simulink model "UAV_Task3"  (R2024b)
settings: Solver=VariableStepAuto  StartTime=0  StopTime=200  RelTol=1e-5  AbsTol=1e-5
values from neighbouring files (symbols this model uses):
  adaptiveActivation = 1    [Simplified_UAV_Task3_main.m]    (also in newUAV_Task3_main.m)
  B_p = 1/UAV.m    [Simplified_UAV_Task3_main.m]    (also in newUAV_Task3_main.m)
  F2plus = F2'*pinv(F2*F2')    [Simplified_UAV_Task3_main.m]    (also in newUAV_Task3_main.m)
  Gamma_a = 1*[1 1 1 1]'    [Simplified_UAV_Task3_main.m]    (also in newUAV_Task3_main.m = 2*[1 1 1 1]')
  gravityInAdaptiveController = 1    [Simplified_UAV_Task3_main.m]    (also in newUAV_Task3_main.m)
  k_f = 0.3379e-6    (= 3.379e-07)    [Simplified_UAV_Task3_main.m]    (also in newUAV_Task3_main.m)
  L = 10    [Simplified_UAV_Task3_main.m]    (also in newUAV_Task3_main.m)
  lambda_0 = 1    [Simplified_UAV_Task3_main.m]    (also in newUAV_Task3_main.m)
  Omega_0 = [1500 1500 1500 1500]'    [Simplified_UAV_Task3_main.m]    (also in newUAV_Task3_main.m)
  omegab_0 = [0; 0; 0]    [Simplified_UAV_Task3_main.m]    (also in newUAV_Task3_main.m)
  p_0 = [0; 0; 0]    [Simplified_UAV_Task3_main.m]    (also in newUAV_Task3_main.m)
  PO = 1    [Simplified_UAV_Task3_main.m]    (also in newUAV_Task3_main.m)
  q_0 = eul2quat([0, 0, 0]*degToRad,'ZYX')'    [Simplified_UAV_Task3_main.m]    (also in newUAV_Task3_main.m)
  scenario = 2    [Simplified_UAV_Task3_main.m]    (also in newUAV_Task3_main.m)
  theta_0 = [0.07;0.07;0.1]    [Simplified_UAV_Task3_main.m]    (also in newUAV_Task3_main.m)
  vb_0 = [0; 0; 0]    [Simplified_UAV_Task3_main.m]    (also in newUAV_Task3_main.m)
undefined symbols (not defined in the file or in its folder): adaptive_controller, ctrl, D_fv_i, dyn, e_3, epsilon_PO, fw_params_fc, g, Gamma_a_scalar, lambda_i, par, pos, pos_pp, projection_operator, targetParams, theta_M, UAV, v_M, vel, vel_pp
libraries: slpidlib x22, matrix_library x6, aerolibutil x2, uavutilslib x1
(part 3 of 4)

== system UAV_Task3/Position Controller/Velocity controller (Dyn) ==
  e_v : Inport
  Demux : Demux  Outputs=3
  Mux : Mux  Inputs=3
  PID Controller vx : slpidlib/PID Controller  Controller=PI  Form=Parallel  TimeDomain=Continuous-time  UseExternalTs=off  SampleTime=-1  IntegratorMethod=Forward Euler  FilterMethod=Forward Euler  ControllerParametersSource=internal  P=ctrl.Kv(1,1)  I=ctrl.Kiv(1,1)  UseKiTs=off  D=0  UseExternalDerivativeSource=off  N=100  UseFilter=on  TunerSelectOption=Transfer Function Based (PID Tuner App)  InitialConditionSource=internal  InitialConditionForIntegrator=0  InitialConditionForFilter=0  DifferentiatorICPrevScaledInput=0  ExternalReset=none  TrackingMode=off  Kt=1  LimitOutput=off  SatLimitsSource=internal  UpperSaturationLimit=inf  LowerSaturationLimit=-inf  LinearizeAsGain=on  AntiWindupMode=none  Kb=1  LimitIntegrator=off  UpperIntegratorSaturationLimit=inf  LowerIntegratorSaturationLimit=-inf  POutMin=[]  POutMax=[]  IOutMin=[]  IOutMax=[]  DOutMin=[]  DOutMax=[]  NOutMin=[]  NOutMax=[]  SumOutMin=[]  SumOutMax=[]  SaturationOutMin=[]  SaturationOutMax=[]  PParamMin=[]  PParamMax=[]  IParamMin=[]  IParamMax=[]  DParamMin=[]  DParamMax=[]  NParamMin=[]  NParamMax=[]  KbParamMin=[]  KbParamMax=[]  KtParamMin=[]  KtParamMax=[]  KbOutMin=[]  KbOutMax=[]  KtOutMin=[]  KtOutMax=[]  IntegratorOutMin=[]  IntegratorOutMax=[]  FilterOutMin=[]  FilterOutMax=[]  SumI1OutMin=[]  SumI1OutMax=[]  SumI2OutMin=[]  SumI2OutMax=[]  SumI3OutMin=[]  SumI3OutMax=[]  SumI4OutMin=[]  SumI4OutMax=[]  SumDOutMin=[]  SumDOutMax=[]  DifferentiatorOutMin=[]  DifferentiatorOutMax=[]  FilterDiffOutCoefMin=[]  FilterDiffOutCoefMax=[]  ReciprocalOutMin=[]  ReciprocalOutMax=[]  SumDenOutMin=[]  SumDenOutMax=[]  SumNumOutMin=[]  SumNumOutMax=[]  DivideOutMin=[]  DivideOutMax=[]  UdiffTsProdOutMin=[]  UdiffTsProdOutMax=[]  NTsProdOutMin=[]  NTsProdOutMax=[]  UintegralTsProdOutMin=[]  UintegralTsProdOutMax=[]  UngainTsProdOutMin=[]  UngainTsProdOutMax=[]  ClampingZeroOutDataTypeStr=Inherit: Inherit via back propagation  ClampingZeroOutMin=[]  ClampingZeroOutMax=[]  FilterDenConstantOutDataTypeStr=Inherit: Inherit via back propagation  FilterDenConstantOutMin=[]  FilterDenConstantOutMax=[]  PCopyOutDataTypeStr=Inherit: Inherit via back propagation  PCopyOutMin=[]  PCopyOutMax=[]  NCopyOutDataTypeStr=Inherit: Inherit via back propagation  NCopyOutMin=[]  NCopyOutMax=[]  IntegratorContinuousStateAttributes=''  IntegratorStateMustResolveToSignalObject=off  IntegratorRTWStateStorageClass=Auto  FilterContinuousStateAttributes=''  FilterStateMustResolveToSignalObject=off  FilterRTWStateStorageClass=Auto  ParallelPVariant=InternalParameters  IdealPVariant=Disabled  IVariant=InternalParameters  DVariant=Disabled  IntegratorVariant=Continuous  SatVariant=Disabled  AWVariant=Passthrough  PCopyVariant=Disabled  TRVariant=Disabled  FdbkBlocksVariant=Forward  IdealPFdbkVariant=Disabled  SatFdbkVariant=Disabled  DerivativeFilterVariant=Disabled  NVariant=Disabled  NCopyVariant=Disabled_SignalSpec  FilterICVariant=Disabled  IntegratorICVariant=InternalICs  ExternalResetVariant=Disabled  TRSumVariant=Passthrough  SumFdbkVariant=Disabled  SumVariant=Sum_PI  TsampFilterVariant=InternalTs  TsampNgainVariant=Passthrough  TsampIntegralVariant=Disabled_SignalSpec  ExternalSaturationOutDataTypeStr=Inherit: Same as second input  DerivativeSourceVariant=Disabled  PreIntVariant=InternalPreInt
  PID Controller vy : slpidlib/PID Controller  Controller=PI  Form=Parallel  TimeDomain=Continuous-time  UseExternalTs=off  SampleTime=-1  IntegratorMethod=Forward Euler  FilterMethod=Forward Euler  ControllerParametersSource=internal  P=ctrl.Kv(2,2)  I=ctrl.Kiv(2,2)  UseKiTs=off  D=0  UseExternalDerivativeSource=off  N=100  UseFilter=on  TunerSelectOption=Transfer Function Based (PID Tuner App)  InitialConditionSource=internal  InitialConditionForIntegrator=0  InitialConditionForFilter=0  DifferentiatorICPrevScaledInput=0  ExternalReset=none  TrackingMode=off  Kt=1  LimitOutput=off  SatLimitsSource=internal  UpperSaturationLimit=inf  LowerSaturationLimit=-inf  LinearizeAsGain=on  AntiWindupMode=none  Kb=1  LimitIntegrator=off  UpperIntegratorSaturationLimit=inf  LowerIntegratorSaturationLimit=-inf  POutMin=[]  POutMax=[]  IOutMin=[]  IOutMax=[]  DOutMin=[]  DOutMax=[]  NOutMin=[]  NOutMax=[]  SumOutMin=[]  SumOutMax=[]  SaturationOutMin=[]  SaturationOutMax=[]  PParamMin=[]  PParamMax=[]  IParamMin=[]  IParamMax=[]  DParamMin=[]  DParamMax=[]  NParamMin=[]  NParamMax=[]  KbParamMin=[]  KbParamMax=[]  KtParamMin=[]  KtParamMax=[]  KbOutMin=[]  KbOutMax=[]  KtOutMin=[]  KtOutMax=[]  IntegratorOutMin=[]  IntegratorOutMax=[]  FilterOutMin=[]  FilterOutMax=[]  SumI1OutMin=[]  SumI1OutMax=[]  SumI2OutMin=[]  SumI2OutMax=[]  SumI3OutMin=[]  SumI3OutMax=[]  SumI4OutMin=[]  SumI4OutMax=[]  SumDOutMin=[]  SumDOutMax=[]  DifferentiatorOutMin=[]  DifferentiatorOutMax=[]  FilterDiffOutCoefMin=[]  FilterDiffOutCoefMax=[]  ReciprocalOutMin=[]  ReciprocalOutMax=[]  SumDenOutMin=[]  SumDenOutMax=[]  SumNumOutMin=[]  SumNumOutMax=[]  DivideOutMin=[]  DivideOutMax=[]  UdiffTsProdOutMin=[]  UdiffTsProdOutMax=[]  NTsProdOutMin=[]  NTsProdOutMax=[]  UintegralTsProdOutMin=[]  UintegralTsProdOutMax=[]  UngainTsProdOutMin=[]  UngainTsProdOutMax=[]  ClampingZeroOutDataTypeStr=Inherit: Inherit via back propagation  ClampingZeroOutMin=[]  ClampingZeroOutMax=[]  FilterDenConstantOutDataTypeStr=Inherit: Inherit via back propagation  FilterDenConstantOutMin=[]  FilterDenConstantOutMax=[]  PCopyOutDataTypeStr=Inherit: Inherit via back propagation  PCopyOutMin=[]  PCopyOutMax=[]  NCopyOutDataTypeStr=Inherit: Inherit via back propagation  NCopyOutMin=[]  NCopyOutMax=[]  IntegratorContinuousStateAttributes=''  IntegratorStateMustResolveToSignalObject=off  IntegratorRTWStateStorageClass=Auto  FilterContinuousStateAttributes=''  FilterStateMustResolveToSignalObject=off  FilterRTWStateStorageClass=Auto  ParallelPVariant=InternalParameters  IdealPVariant=Disabled  IVariant=InternalParameters  DVariant=Disabled  IntegratorVariant=Continuous  SatVariant=Disabled  AWVariant=Passthrough  PCopyVariant=Disabled  TRVariant=Disabled  FdbkBlocksVariant=Forward  IdealPFdbkVariant=Disabled  SatFdbkVariant=Disabled  DerivativeFilterVariant=Disabled  NVariant=Disabled  NCopyVariant=Disabled_SignalSpec  FilterICVariant=Disabled  IntegratorICVariant=InternalICs  ExternalResetVariant=Disabled  TRSumVariant=Passthrough  SumFdbkVariant=Disabled  SumVariant=Sum_PI  TsampFilterVariant=InternalTs  TsampNgainVariant=Passthrough  TsampIntegralVariant=Disabled_SignalSpec  ExternalSaturationOutDataTypeStr=Inherit: Same as second input  DerivativeSourceVariant=Disabled  PreIntVariant=InternalPreInt
  PID Controller vz : slpidlib/PID Controller  Controller=PI  Form=Parallel  TimeDomain=Continuous-time  UseExternalTs=off  SampleTime=-1  IntegratorMethod=Forward Euler  FilterMethod=Forward Euler  ControllerParametersSource=internal  P=ctrl.Kv(3,3)  I=ctrl.Kiv(3,3)  UseKiTs=off  D=0  UseExternalDerivativeSource=off  N=100  UseFilter=on  TunerSelectOption=Transfer Function Based (PID Tuner App)  InitialConditionSource=internal  InitialConditionForIntegrator=0  InitialConditionForFilter=0  DifferentiatorICPrevScaledInput=0  ExternalReset=none  TrackingMode=off  Kt=1  LimitOutput=off  SatLimitsSource=internal  UpperSaturationLimit=inf  LowerSaturationLimit=-inf  LinearizeAsGain=on  AntiWindupMode=none  Kb=1  LimitIntegrator=off  UpperIntegratorSaturationLimit=inf  LowerIntegratorSaturationLimit=-inf  POutMin=[]  POutMax=[]  IOutMin=[]  IOutMax=[]  DOutMin=[]  DOutMax=[]  NOutMin=[]  NOutMax=[]  SumOutMin=[]  SumOutMax=[]  SaturationOutMin=[]  SaturationOutMax=[]  PParamMin=[]  PParamMax=[]  IParamMin=[]  IParamMax=[]  DParamMin=[]  DParamMax=[]  NParamMin=[]  NParamMax=[]  KbParamMin=[]  KbParamMax=[]  KtParamMin=[]  KtParamMax=[]  KbOutMin=[]  KbOutMax=[]  KtOutMin=[]  KtOutMax=[]  IntegratorOutMin=[]  IntegratorOutMax=[]  FilterOutMin=[]  FilterOutMax=[]  SumI1OutMin=[]  SumI1OutMax=[]  SumI2OutMin=[]  SumI2OutMax=[]  SumI3OutMin=[]  SumI3OutMax=[]  SumI4OutMin=[]  SumI4OutMax=[]  SumDOutMin=[]  SumDOutMax=[]  DifferentiatorOutMin=[]  DifferentiatorOutMax=[]  FilterDiffOutCoefMin=[]  FilterDiffOutCoefMax=[]  ReciprocalOutMin=[]  ReciprocalOutMax=[]  SumDenOutMin=[]  SumDenOutMax=[]  SumNumOutMin=[]  SumNumOutMax=[]  DivideOutMin=[]  DivideOutMax=[]  UdiffTsProdOutMin=[]  UdiffTsProdOutMax=[]  NTsProdOutMin=[]  NTsProdOutMax=[]  UintegralTsProdOutMin=[]  UintegralTsProdOutMax=[]  UngainTsProdOutMin=[]  UngainTsProdOutMax=[]  ClampingZeroOutDataTypeStr=Inherit: Inherit via back propagation  ClampingZeroOutMin=[]  ClampingZeroOutMax=[]  FilterDenConstantOutDataTypeStr=Inherit: Inherit via back propagation  FilterDenConstantOutMin=[]  FilterDenConstantOutMax=[]  PCopyOutDataTypeStr=Inherit: Inherit via back propagation  PCopyOutMin=[]  PCopyOutMax=[]  NCopyOutDataTypeStr=Inherit: Inherit via back propagation  NCopyOutMin=[]  NCopyOutMax=[]  IntegratorContinuousStateAttributes=''  IntegratorStateMustResolveToSignalObject=off  IntegratorRTWStateStorageClass=Auto  FilterContinuousStateAttributes=''  FilterStateMustResolveToSignalObject=off  FilterRTWStateStorageClass=Auto  ParallelPVariant=InternalParameters  IdealPVariant=Disabled  IVariant=InternalParameters  DVariant=Disabled  IntegratorVariant=Continuous  SatVariant=Disabled  AWVariant=Passthrough  PCopyVariant=Disabled  TRVariant=Disabled  FdbkBlocksVariant=Forward  IdealPFdbkVariant=Disabled  SatFdbkVariant=Disabled  DerivativeFilterVariant=Disabled  NVariant=Disabled  NCopyVariant=Disabled_SignalSpec  FilterICVariant=Disabled  IntegratorICVariant=InternalICs  ExternalResetVariant=Disabled  TRSumVariant=Passthrough  SumFdbkVariant=Disabled  SumVariant=Sum_PI  TsampFilterVariant=InternalTs  TsampNgainVariant=Passthrough  TsampIntegralVariant=Disabled_SignalSpec  ExternalSaturationOutDataTypeStr=Inherit: Same as second input  DerivativeSourceVariant=Disabled  PreIntVariant=InternalPreInt
  2 : Outport
  wires:
  PID Controller vy/1 -> Mux/2
  Demux/2 -> PID Controller vy/1
  e_v/1 -> Demux/1
  Demux/3 -> PID Controller vz/1
  PID Controller vx/1 -> Mux/1
  PID Controller vz/1 -> Mux/3
  Demux/1 -> PID Controller vx/1
  Mux/1 -> 2/1

== system UAV_Task3/ATTITUDE CONTROLLER/Attitude dynamics FF/Feedback controller ==
  e_omega : Inport
  Demux : Demux  Outputs=3
  Mux : Mux  Inputs=3
  PID Controller p : slpidlib/PID Controller  Controller=PI  Form=Parallel  TimeDomain=Continuous-time  UseExternalTs=off  SampleTime=-1  IntegratorMethod=Forward Euler  FilterMethod=Forward Euler  ControllerParametersSource=internal  P=dyn.Kp(1,1)  I=dyn.Ki(1,1)  UseKiTs=off  D=0  UseExternalDerivativeSource=off  N=100  UseFilter=on  TunerSelectOption=Transfer Function Based (PID Tuner App)  InitialConditionSource=internal  InitialConditionForIntegrator=0  InitialConditionForFilter=0  DifferentiatorICPrevScaledInput=0  ExternalReset=none  TrackingMode=off  Kt=1  LimitOutput=off  SatLimitsSource=internal  UpperSaturationLimit=inf  LowerSaturationLimit=-inf  LinearizeAsGain=on  AntiWindupMode=none  Kb=1  LimitIntegrator=off  UpperIntegratorSaturationLimit=inf  LowerIntegratorSaturationLimit=-inf  POutMin=[]  POutMax=[]  IOutMin=[]  IOutMax=[]  DOutMin=[]  DOutMax=[]  NOutMin=[]  NOutMax=[]  SumOutMin=[]  SumOutMax=[]  SaturationOutMin=[]  SaturationOutMax=[]  PParamMin=[]  PParamMax=[]  IParamMin=[]  IParamMax=[]  DParamMin=[]  DParamMax=[]  NParamMin=[]  NParamMax=[]  KbParamMin=[]  KbParamMax=[]  KtParamMin=[]  KtParamMax=[]  KbOutMin=[]  KbOutMax=[]  KtOutMin=[]  KtOutMax=[]  IntegratorOutMin=[]  IntegratorOutMax=[]  FilterOutMin=[]  FilterOutMax=[]  SumI1OutMin=[]  SumI1OutMax=[]  SumI2OutMin=[]  SumI2OutMax=[]  SumI3OutMin=[]  SumI3OutMax=[]  SumI4OutMin=[]  SumI4OutMax=[]  SumDOutMin=[]  SumDOutMax=[]  DifferentiatorOutMin=[]  DifferentiatorOutMax=[]  FilterDiffOutCoefMin=[]  FilterDiffOutCoefMax=[]  ReciprocalOutMin=[]  ReciprocalOutMax=[]  SumDenOutMin=[]  SumDenOutMax=[]  SumNumOutMin=[]  SumNumOutMax=[]  DivideOutMin=[]  DivideOutMax=[]  UdiffTsProdOutMin=[]  UdiffTsProdOutMax=[]  NTsProdOutMin=[]  NTsProdOutMax=[]  UintegralTsProdOutMin=[]  UintegralTsProdOutMax=[]  UngainTsProdOutMin=[]  UngainTsProdOutMax=[]  ClampingZeroOutDataTypeStr=Inherit: Inherit via back propagation  ClampingZeroOutMin=[]  ClampingZeroOutMax=[]  FilterDenConstantOutDataTypeStr=Inherit: Inherit via back propagation  FilterDenConstantOutMin=[]  FilterDenConstantOutMax=[]  PCopyOutDataTypeStr=Inherit: Inherit via back propagation  PCopyOutMin=[]  PCopyOutMax=[]  NCopyOutDataTypeStr=Inherit: Inherit via back propagation  NCopyOutMin=[]  NCopyOutMax=[]  IntegratorContinuousStateAttributes=''  IntegratorStateMustResolveToSignalObject=off  IntegratorRTWStateStorageClass=Auto  FilterContinuousStateAttributes=''  FilterStateMustResolveToSignalObject=off  FilterRTWStateStorageClass=Auto  ParallelPVariant=InternalParameters  IdealPVariant=Disabled  IVariant=InternalParameters  DVariant=Disabled  IntegratorVariant=Continuous  SatVariant=Disabled  AWVariant=Passthrough  PCopyVariant=Disabled  TRVariant=Disabled  FdbkBlocksVariant=Forward  IdealPFdbkVariant=Disabled  SatFdbkVariant=Disabled  DerivativeFilterVariant=Disabled  NVariant=Disabled  NCopyVariant=Disabled_SignalSpec  FilterICVariant=Disabled  IntegratorICVariant=InternalICs  ExternalResetVariant=Disabled  TRSumVariant=Passthrough  SumFdbkVariant=Disabled  SumVariant=Sum_PI  TsampFilterVariant=InternalTs  TsampNgainVariant=Passthrough  TsampIntegralVariant=Disabled_SignalSpec  ExternalSaturationOutDataTypeStr=Inherit: Same as second input  DerivativeSourceVariant=Disabled  PreIntVariant=InternalPreInt
  PID Controller q : slpidlib/PID Controller  Controller=PI  Form=Parallel  TimeDomain=Continuous-time  UseExternalTs=off  SampleTime=-1  IntegratorMethod=Forward Euler  FilterMethod=Forward Euler  ControllerParametersSource=internal  P=dyn.Kp(2,2)  I=dyn.Ki(2,2)  UseKiTs=off  D=0  UseExternalDerivativeSource=off  N=100  UseFilter=on  TunerSelectOption=Transfer Function Based (PID Tuner App)  InitialConditionSource=internal  InitialConditionForIntegrator=0  InitialConditionForFilter=0  DifferentiatorICPrevScaledInput=0  ExternalReset=none  TrackingMode=off  Kt=1  LimitOutput=off  SatLimitsSource=internal  UpperSaturationLimit=inf  LowerSaturationLimit=-inf  LinearizeAsGain=on  AntiWindupMode=none  Kb=1  LimitIntegrator=off  UpperIntegratorSaturationLimit=inf  LowerIntegratorSaturationLimit=-inf  POutMin=[]  POutMax=[]  IOutMin=[]  IOutMax=[]  DOutMin=[]  DOutMax=[]  NOutMin=[]  NOutMax=[]  SumOutMin=[]  SumOutMax=[]  SaturationOutMin=[]  SaturationOutMax=[]  PParamMin=[]  PParamMax=[]  IParamMin=[]  IParamMax=[]  DParamMin=[]  DParamMax=[]  NParamMin=[]  NParamMax=[]  KbParamMin=[]  KbParamMax=[]  KtParamMin=[]  KtParamMax=[]  KbOutMin=[]  KbOutMax=[]  KtOutMin=[]  KtOutMax=[]  IntegratorOutMin=[]  IntegratorOutMax=[]  FilterOutMin=[]  FilterOutMax=[]  SumI1OutMin=[]  SumI1OutMax=[]  SumI2OutMin=[]  SumI2OutMax=[]  SumI3OutMin=[]  SumI3OutMax=[]  SumI4OutMin=[]  SumI4OutMax=[]  SumDOutMin=[]  SumDOutMax=[]  DifferentiatorOutMin=[]  DifferentiatorOutMax=[]  FilterDiffOutCoefMin=[]  FilterDiffOutCoefMax=[]  ReciprocalOutMin=[]  ReciprocalOutMax=[]  SumDenOutMin=[]  SumDenOutMax=[]  SumNumOutMin=[]  SumNumOutMax=[]  DivideOutMin=[]  DivideOutMax=[]  UdiffTsProdOutMin=[]  UdiffTsProdOutMax=[]  NTsProdOutMin=[]  NTsProdOutMax=[]  UintegralTsProdOutMin=[]  UintegralTsProdOutMax=[]  UngainTsProdOutMin=[]  UngainTsProdOutMax=[]  ClampingZeroOutDataTypeStr=Inherit: Inherit via back propagation  ClampingZeroOutMin=[]  ClampingZeroOutMax=[]  FilterDenConstantOutDataTypeStr=Inherit: Inherit via back propagation  FilterDenConstantOutMin=[]  FilterDenConstantOutMax=[]  PCopyOutDataTypeStr=Inherit: Inherit via back propagation  PCopyOutMin=[]  PCopyOutMax=[]  NCopyOutDataTypeStr=Inherit: Inherit via back propagation  NCopyOutMin=[]  NCopyOutMax=[]  IntegratorContinuousStateAttributes=''  IntegratorStateMustResolveToSignalObject=off  IntegratorRTWStateStorageClass=Auto  FilterContinuousStateAttributes=''  FilterStateMustResolveToSignalObject=off  FilterRTWStateStorageClass=Auto  ParallelPVariant=InternalParameters  IdealPVariant=Disabled  IVariant=InternalParameters  DVariant=Disabled  IntegratorVariant=Continuous  SatVariant=Disabled  AWVariant=Passthrough  PCopyVariant=Disabled  TRVariant=Disabled  FdbkBlocksVariant=Forward  IdealPFdbkVariant=Disabled  SatFdbkVariant=Disabled  DerivativeFilterVariant=Disabled  NVariant=Disabled  NCopyVariant=Disabled_SignalSpec  FilterICVariant=Disabled  IntegratorICVariant=InternalICs  ExternalResetVariant=Disabled  TRSumVariant=Passthrough  SumFdbkVariant=Disabled  SumVariant=Sum_PI  TsampFilterVariant=InternalTs  TsampNgainVariant=Passthrough  TsampIntegralVariant=Disabled_SignalSpec  ExternalSaturationOutDataTypeStr=Inherit: Same as second input  DerivativeSourceVariant=Disabled  PreIntVariant=InternalPreInt
  PID Controller r : slpidlib/PID Controller  Controller=PI  Form=Parallel  TimeDomain=Continuous-time  UseExternalTs=off  SampleTime=-1  IntegratorMethod=Forward Euler  FilterMethod=Forward Euler  ControllerParametersSource=internal  P=dyn.Kp(3,3)  I=dyn.Ki(3,3)  UseKiTs=off  D=0  UseExternalDerivativeSource=off  N=100  UseFilter=on  TunerSelectOption=Transfer Function Based (PID Tuner App)  InitialConditionSource=internal  InitialConditionForIntegrator=0  InitialConditionForFilter=0  DifferentiatorICPrevScaledInput=0  ExternalReset=none  TrackingMode=off  Kt=1  LimitOutput=off  SatLimitsSource=internal  UpperSaturationLimit=inf  LowerSaturationLimit=-inf  LinearizeAsGain=on  AntiWindupMode=none  Kb=1  LimitIntegrator=off  UpperIntegratorSaturationLimit=inf  LowerIntegratorSaturationLimit=-inf  POutMin=[]  POutMax=[]  IOutMin=[]  IOutMax=[]  DOutMin=[]  DOutMax=[]  NOutMin=[]  NOutMax=[]  SumOutMin=[]  SumOutMax=[]  SaturationOutMin=[]  SaturationOutMax=[]  PParamMin=[]  PParamMax=[]  IParamMin=[]  IParamMax=[]  DParamMin=[]  DParamMax=[]  NParamMin=[]  NParamMax=[]  KbParamMin=[]  KbParamMax=[]  KtParamMin=[]  KtParamMax=[]  KbOutMin=[]  KbOutMax=[]  KtOutMin=[]  KtOutMax=[]  IntegratorOutMin=[]  IntegratorOutMax=[]  FilterOutMin=[]  FilterOutMax=[]  SumI1OutMin=[]  SumI1OutMax=[]  SumI2OutMin=[]  SumI2OutMax=[]  SumI3OutMin=[]  SumI3OutMax=[]  SumI4OutMin=[]  SumI4OutMax=[]  SumDOutMin=[]  SumDOutMax=[]  DifferentiatorOutMin=[]  DifferentiatorOutMax=[]  FilterDiffOutCoefMin=[]  FilterDiffOutCoefMax=[]  ReciprocalOutMin=[]  ReciprocalOutMax=[]  SumDenOutMin=[]  SumDenOutMax=[]  SumNumOutMin=[]  SumNumOutMax=[]  DivideOutMin=[]  DivideOutMax=[]  UdiffTsProdOutMin=[]  UdiffTsProdOutMax=[]  NTsProdOutMin=[]  NTsProdOutMax=[]  UintegralTsProdOutMin=[]  UintegralTsProdOutMax=[]  UngainTsProdOutMin=[]  UngainTsProdOutMax=[]  ClampingZeroOutDataTypeStr=Inherit: Inherit via back propagation  ClampingZeroOutMin=[]  ClampingZeroOutMax=[]  FilterDenConstantOutDataTypeStr=Inherit: Inherit via back propagation  FilterDenConstantOutMin=[]  FilterDenConstantOutMax=[]  PCopyOutDataTypeStr=Inherit: Inherit via back propagation  PCopyOutMin=[]  PCopyOutMax=[]  NCopyOutDataTypeStr=Inherit: Inherit via back propagation  NCopyOutMin=[]  NCopyOutMax=[]  IntegratorContinuousStateAttributes=''  IntegratorStateMustResolveToSignalObject=off  IntegratorRTWStateStorageClass=Auto  FilterContinuousStateAttributes=''  FilterStateMustResolveToSignalObject=off  FilterRTWStateStorageClass=Auto  ParallelPVariant=InternalParameters  IdealPVariant=Disabled  IVariant=InternalParameters  DVariant=Disabled  IntegratorVariant=Continuous  SatVariant=Disabled  AWVariant=Passthrough  PCopyVariant=Disabled  TRVariant=Disabled  FdbkBlocksVariant=Forward  IdealPFdbkVariant=Disabled  SatFdbkVariant=Disabled  DerivativeFilterVariant=Disabled  NVariant=Disabled  NCopyVariant=Disabled_SignalSpec  FilterICVariant=Disabled  IntegratorICVariant=InternalICs  ExternalResetVariant=Disabled  TRSumVariant=Passthrough  SumFdbkVariant=Disabled  SumVariant=Sum_PI  TsampFilterVariant=InternalTs  TsampNgainVariant=Passthrough  TsampIntegralVariant=Disabled_SignalSpec  ExternalSaturationOutDataTypeStr=Inherit: Same as second input  DerivativeSourceVariant=Disabled  PreIntVariant=InternalPreInt
  tau_fbk : Outport
  wires:
  Mux/1 -> tau_fbk/1
  Demux/1 -> PID Controller p/1
  PID Controller r/1 -> Mux/3
  PID Controller p/1 -> Mux/1
  Demux/3 -> PID Controller r/1
  e_omega/1 -> Demux/1
  Demux/2 -> PID Controller q/1
  PID Controller q/1 -> Mux/2

== system UAV_Task3/POSITION + ADAPTIVE CONTROLLER/POSITION CONTROLLER/Position controller ==
  p : Inport
  p_d : Inport  Port=2
  v_d : Inport  Port=3
  a_d : Inport  Port=4
  v : Inport  Port=5
  MATLAB Function1 : MATLAB Function  TreatAsAtomicUnit=on
  " v_c" : Outport
  " a_c" : Outport  Port=2
  wires:
  MATLAB Function1/1(v_c) -> " v_c"/1
  a_d/1 -> MATLAB Function1/5(a_d)
  p/1 -> MATLAB Function1/1(p)
  p_d/1 -> MATLAB Function1/3(p_d)  "p_d"
  v_d/1 -> MATLAB Function1/4(v_d)
  v/1 -> MATLAB Function1/2(v)
  MATLAB Function1/2(a_c) -> " a_c"/1

== system UAV_Task3/POSITION + ADAPTIVE CONTROLLER/POSITION CONTROLLER/Velocity Controller ==
  v : Inport
  v_c : Inport  Port=2
  a_c : Inport  Port=3
  Demux : Demux  Outputs=3
  Gain : Gain  Gain=UAV.m
  Mux : Mux  Inputs=3
  PID Controller1 : slpidlib/PID Controller  Controller=PI  Form=Parallel  TimeDomain=Continuous-time  UseExternalTs=off  SampleTime=-1  IntegratorMethod=Forward Euler  FilterMethod=Forward Euler  ControllerParametersSource=internal  P=vel.Kp(2,2)  I=vel.Ki(2,2)  UseKiTs=off  D=0  UseExternalDerivativeSource=off  N=100  UseFilter=on  TunerSelectOption=Transfer Function Based (PID Tuner App)  InitialConditionSource=internal  InitialConditionForIntegrator=0  InitialConditionForFilter=0  DifferentiatorICPrevScaledInput=0  ExternalReset=none  TrackingMode=off  Kt=1  LimitOutput=off  SatLimitsSource=internal  UpperSaturationLimit=inf  LowerSaturationLimit=-inf  LinearizeAsGain=on  AntiWindupMode=none  Kb=1  LimitIntegrator=off  UpperIntegratorSaturationLimit=inf  LowerIntegratorSaturationLimit=-inf  POutMin=[]  POutMax=[]  IOutMin=[]  IOutMax=[]  DOutMin=[]  DOutMax=[]  NOutMin=[]  NOutMax=[]  SumOutMin=[]  SumOutMax=[]  SaturationOutMin=[]  SaturationOutMax=[]  PParamMin=[]  PParamMax=[]  IParamMin=[]  IParamMax=[]  DParamMin=[]  DParamMax=[]  NParamMin=[]  NParamMax=[]  KbParamMin=[]  KbParamMax=[]  KtParamMin=[]  KtParamMax=[]  KbOutMin=[]  KbOutMax=[]  KtOutMin=[]  KtOutMax=[]  IntegratorOutMin=[]  IntegratorOutMax=[]  FilterOutMin=[]  FilterOutMax=[]  SumI1OutMin=[]  SumI1OutMax=[]  SumI2OutMin=[]  SumI2OutMax=[]  SumI3OutMin=[]  SumI3OutMax=[]  SumI4OutMin=[]  SumI4OutMax=[]  SumDOutMin=[]  SumDOutMax=[]  DifferentiatorOutMin=[]  DifferentiatorOutMax=[]  FilterDiffOutCoefMin=[]  FilterDiffOutCoefMax=[]  ReciprocalOutMin=[]  ReciprocalOutMax=[]  SumDenOutMin=[]  SumDenOutMax=[]  SumNumOutMin=[]  SumNumOutMax=[]  DivideOutMin=[]  DivideOutMax=[]  UdiffTsProdOutMin=[]  UdiffTsProdOutMax=[]  NTsProdOutMin=[]  NTsProdOutMax=[]  UintegralTsProdOutMin=[]  UintegralTsProdOutMax=[]  UngainTsProdOutMin=[]  UngainTsProdOutMax=[]  ClampingZeroOutDataTypeStr=Inherit: Inherit via back propagation  ClampingZeroOutMin=[]  ClampingZeroOutMax=[]  FilterDenConstantOutDataTypeStr=Inherit: Inherit via back propagation  FilterDenConstantOutMin=[]  FilterDenConstantOutMax=[]  PCopyOutDataTypeStr=Inherit: Inherit via back propagation  PCopyOutMin=[]  PCopyOutMax=[]  NCopyOutDataTypeStr=Inherit: Inherit via back propagation  NCopyOutMin=[]  NCopyOutMax=[]  IntegratorContinuousStateAttributes=''  IntegratorStateMustResolveToSignalObject=off  IntegratorRTWStateStorageClass=Auto  FilterContinuousStateAttributes=''  FilterStateMustResolveToSignalObject=off  FilterRTWStateStorageClass=Auto  ParallelPVariant=InternalParameters  IdealPVariant=Disabled  IVariant=InternalParameters  DVariant=Disabled  IntegratorVariant=Continuous  SatVariant=Disabled  AWVariant=Passthrough  PCopyVariant=Disabled  TRVariant=Disabled  FdbkBlocksVariant=Forward  IdealPFdbkVariant=Disabled  SatFdbkVariant=Disabled  DerivativeFilterVariant=Disabled  NVariant=Disabled  NCopyVariant=Disabled_SignalSpec  FilterICVariant=Disabled  IntegratorICVariant=InternalICs  ExternalResetVariant=Disabled  TRSumVariant=Passthrough  SumFdbkVariant=Disabled  SumVariant=Sum_PI  TsampFilterVariant=InternalTs  TsampNgainVariant=Passthrough  TsampIntegralVariant=Disabled_SignalSpec  ExternalSaturationOutDataTypeStr=Inherit: Same as second input  DerivativeSourceVariant=Disabled  PreIntVariant=InternalPreInt
  PID Controller2 : slpidlib/PID Controller  Controller=PI  Form=Parallel  TimeDomain=Continuous-time  UseExternalTs=off  SampleTime=-1  IntegratorMethod=Forward Euler  FilterMethod=Forward Euler  ControllerParametersSource=internal  P=vel.Kp(3,3)  I=vel.Ki(3,3)  UseKiTs=off  D=0  UseExternalDerivativeSource=off  N=100  UseFilter=on  TunerSelectOption=Transfer Function Based (PID Tuner App)  InitialConditionSource=internal  InitialConditionForIntegrator=0  InitialConditionForFilter=0  DifferentiatorICPrevScaledInput=0  ExternalReset=none  TrackingMode=off  Kt=1  LimitOutput=off  SatLimitsSource=internal  UpperSaturationLimit=inf  LowerSaturationLimit=-inf  LinearizeAsGain=on  AntiWindupMode=none  Kb=1  LimitIntegrator=off  UpperIntegratorSaturationLimit=inf  LowerIntegratorSaturationLimit=-inf  POutMin=[]  POutMax=[]  IOutMin=[]  IOutMax=[]  DOutMin=[]  DOutMax=[]  NOutMin=[]  NOutMax=[]  SumOutMin=[]  SumOutMax=[]  SaturationOutMin=[]  SaturationOutMax=[]  PParamMin=[]  PParamMax=[]  IParamMin=[]  IParamMax=[]  DParamMin=[]  DParamMax=[]  NParamMin=[]  NParamMax=[]  KbParamMin=[]  KbParamMax=[]  KtParamMin=[]  KtParamMax=[]  KbOutMin=[]  KbOutMax=[]  KtOutMin=[]  KtOutMax=[]  IntegratorOutMin=[]  IntegratorOutMax=[]  FilterOutMin=[]  FilterOutMax=[]  SumI1OutMin=[]  SumI1OutMax=[]  SumI2OutMin=[]  SumI2OutMax=[]  SumI3OutMin=[]  SumI3OutMax=[]  SumI4OutMin=[]  SumI4OutMax=[]  SumDOutMin=[]  SumDOutMax=[]  DifferentiatorOutMin=[]  DifferentiatorOutMax=[]  FilterDiffOutCoefMin=[]  FilterDiffOutCoefMax=[]  ReciprocalOutMin=[]  ReciprocalOutMax=[]  SumDenOutMin=[]  SumDenOutMax=[]  SumNumOutMin=[]  SumNumOutMax=[]  DivideOutMin=[]  DivideOutMax=[]  UdiffTsProdOutMin=[]  UdiffTsProdOutMax=[]  NTsProdOutMin=[]  NTsProdOutMax=[]  UintegralTsProdOutMin=[]  UintegralTsProdOutMax=[]  UngainTsProdOutMin=[]  UngainTsProdOutMax=[]  ClampingZeroOutDataTypeStr=Inherit: Inherit via back propagation  ClampingZeroOutMin=[]  ClampingZeroOutMax=[]  FilterDenConstantOutDataTypeStr=Inherit: Inherit via back propagation  FilterDenConstantOutMin=[]  FilterDenConstantOutMax=[]  PCopyOutDataTypeStr=Inherit: Inherit via back propagation  PCopyOutMin=[]  PCopyOutMax=[]  NCopyOutDataTypeStr=Inherit: Inherit via back propagation  NCopyOutMin=[]  NCopyOutMax=[]  IntegratorContinuousStateAttributes=''  IntegratorStateMustResolveToSignalObject=off  IntegratorRTWStateStorageClass=Auto  FilterContinuousStateAttributes=''  FilterStateMustResolveToSignalObject=off  FilterRTWStateStorageClass=Auto  ParallelPVariant=InternalParameters  IdealPVariant=Disabled  IVariant=InternalParameters  DVariant=Disabled  IntegratorVariant=Continuous  SatVariant=Disabled  AWVariant=Passthrough  PCopyVariant=Disabled  TRVariant=Disabled  FdbkBlocksVariant=Forward  IdealPFdbkVariant=Disabled  SatFdbkVariant=Disabled  DerivativeFilterVariant=Disabled  NVariant=Disabled  NCopyVariant=Disabled_SignalSpec  FilterICVariant=Disabled  IntegratorICVariant=InternalICs  ExternalResetVariant=Disabled  TRSumVariant=Passthrough  SumFdbkVariant=Disabled  SumVariant=Sum_PI  TsampFilterVariant=InternalTs  TsampNgainVariant=Passthrough  TsampIntegralVariant=Disabled_SignalSpec  ExternalSaturationOutDataTypeStr=Inherit: Same as second input  DerivativeSourceVariant=Disabled  PreIntVariant=InternalPreInt
  PID Controller3 : slpidlib/PID Controller  Controller=PI  Form=Parallel  TimeDomain=Continuous-time  UseExternalTs=off  SampleTime=-1  IntegratorMethod=Forward Euler  FilterMethod=Forward Euler  ControllerParametersSource=internal  P=vel.Kp(1,1)  I=vel.Ki(1,1)  UseKiTs=off  D=0  UseExternalDerivativeSource=off  N=100  UseFilter=on  TunerSelectOption=Transfer Function Based (PID Tuner App)  InitialConditionSource=internal  InitialConditionForIntegrator=0  InitialConditionForFilter=0  DifferentiatorICPrevScaledInput=0  ExternalReset=none  TrackingMode=off  Kt=1  LimitOutput=off  SatLimitsSource=internal  UpperSaturationLimit=inf  LowerSaturationLimit=-inf  LinearizeAsGain=on  AntiWindupMode=none  Kb=1  LimitIntegrator=off  UpperIntegratorSaturationLimit=inf  LowerIntegratorSaturationLimit=-inf  POutMin=[]  POutMax=[]  IOutMin=[]  IOutMax=[]  DOutMin=[]  DOutMax=[]  NOutMin=[]  NOutMax=[]  SumOutMin=[]  SumOutMax=[]  SaturationOutMin=[]  SaturationOutMax=[]  PParamMin=[]  PParamMax=[]  IParamMin=[]  IParamMax=[]  DParamMin=[]  DParamMax=[]  NParamMin=[]  NParamMax=[]  KbParamMin=[]  KbParamMax=[]  KtParamMin=[]  KtParamMax=[]  KbOutMin=[]  KbOutMax=[]  KtOutMin=[]  KtOutMax=[]  IntegratorOutMin=[]  IntegratorOutMax=[]  FilterOutMin=[]  FilterOutMax=[]  SumI1OutMin=[]  SumI1OutMax=[]  SumI2OutMin=[]  SumI2OutMax=[]  SumI3OutMin=[]  SumI3OutMax=[]  SumI4OutMin=[]  SumI4OutMax=[]  SumDOutMin=[]  SumDOutMax=[]  DifferentiatorOutMin=[]  DifferentiatorOutMax=[]  FilterDiffOutCoefMin=[]  FilterDiffOutCoefMax=[]  ReciprocalOutMin=[]  ReciprocalOutMax=[]  SumDenOutMin=[]  SumDenOutMax=[]  SumNumOutMin=[]  SumNumOutMax=[]  DivideOutMin=[]  DivideOutMax=[]  UdiffTsProdOutMin=[]  UdiffTsProdOutMax=[]  NTsProdOutMin=[]  NTsProdOutMax=[]  UintegralTsProdOutMin=[]  UintegralTsProdOutMax=[]  UngainTsProdOutMin=[]  UngainTsProdOutMax=[]  ClampingZeroOutDataTypeStr=Inherit: Inherit via back propagation  ClampingZeroOutMin=[]  ClampingZeroOutMax=[]  FilterDenConstantOutDataTypeStr=Inherit: Inherit via back propagation  FilterDenConstantOutMin=[]  FilterDenConstantOutMax=[]  PCopyOutDataTypeStr=Inherit: Inherit via back propagation  PCopyOutMin=[]  PCopyOutMax=[]  NCopyOutDataTypeStr=Inherit: Inherit via back propagation  NCopyOutMin=[]  NCopyOutMax=[]  IntegratorContinuousStateAttributes=''  IntegratorStateMustResolveToSignalObject=off  IntegratorRTWStateStorageClass=Auto  FilterContinuousStateAttributes=''  FilterStateMustResolveToSignalObject=off  FilterRTWStateStorageClass=Auto  ParallelPVariant=InternalParameters  IdealPVariant=Disabled  IVariant=InternalParameters  DVariant=Disabled  IntegratorVariant=Continuous  SatVariant=Disabled  AWVariant=Passthrough  PCopyVariant=Disabled  TRVariant=Disabled  FdbkBlocksVariant=Forward  IdealPFdbkVariant=Disabled  SatFdbkVariant=Disabled  DerivativeFilterVariant=Disabled  NVariant=Disabled  NCopyVariant=Disabled_SignalSpec  FilterICVariant=Disabled  IntegratorICVariant=InternalICs  ExternalResetVariant=Disabled  TRSumVariant=Passthrough  SumFdbkVariant=Disabled  SumVariant=Sum_PI  TsampFilterVariant=InternalTs  TsampNgainVariant=Passthrough  TsampIntegralVariant=Disabled_SignalSpec  ExternalSaturationOutDataTypeStr=Inherit: Same as second input  DerivativeSourceVariant=Disabled  PreIntVariant=InternalPreInt
  Sum : Sum  Inputs=+-
  Sum1 : Sum  Inputs=--+
  "gravity compensation " : Constant  Value=UAV.m*g*e_3
  f_c : Outport
  wires:
  Demux/1 -> PID Controller3/1
  PID Controller1/1 -> Mux/2
  Demux/2 -> PID Controller1/1
  PID Controller2/1 -> Mux/3
  PID Controller3/1 -> Mux/1
  Sum/1 -> Demux/1  "e_v"
  Demux/3 -> PID Controller2/1
  v/1 -> Sum/1
  v_c/1 -> Sum/2
  a_c/1 -> Gain/1
  Sum1/1 -> f_c/1
  Mux/1 -> Sum1/2
  Gain/1 -> Sum1/3
  "gravity compensation "/1 -> Sum1/1

== system UAV_Task3/POSITION + ADAPTIVE CONTROLLER/Subsystem1/Subsystem ==
  v : Inport
  phipT : Inport  Port=2
  lambda_hat : Inport  Port=3
  u : Inport  Port=4
  thetap_hat : Inport  Port=5
  Constant : Constant  Value=[0 0 g]
  Gain : Gain  Gain=1/UAV.m
  Gain1 : Gain  Gain=L
  Integrator : Integrator  InitialCondition=vb_0
  Matrix Multiply : Product  Multiplication=Matrix(*)
  Matrix Multiply1 : Product  Multiplication=Matrix(*)
  Scope : Scope
  Sum : Sum  Inputs=+++
  Sum1 : Sum
  Sum2 : Sum  Inputs=|+-
  v_hat : Outport
  ev : Outport  Port=2
  wires:
  lambda_hat/1 -> Matrix Multiply/1
  u/1 -> Matrix Multiply/2
  phipT/1 -> Matrix Multiply1/1
  thetap_hat/1 -> Matrix Multiply1/2
  Matrix Multiply1/1 -> Sum1/1
  Matrix Multiply/1 -> Sum1/2
  Sum1/1 -> Gain/1
  Constant/1 -> Sum/1
  Gain/1 -> Sum/2
  Sum/1 -> Integrator/1
  Integrator/1 -> Sum2/2, v_hat/1
  v/1 -> Sum2/1
  Sum2/1 -> Scope/1, ev/1, Gain1/1
  Gain1/1 -> Sum/3

== system UAV_Task3/POSITION + ADAPTIVE CONTROLLER/Subsystem1/Subsystem1 ==
  phia : Inport
  ev : Inport  Port=2
  Adaptive Augmentation : Subsystem  Commented=on
  Constant : Constant  Value=Gamma_a_scalar
  Constant1 : Constant  Value=projection_operator
  Gain : Gain  Gain=1/UAV.m
  Integrator : Integrator  InitialCondition=[lambda_i; D_fv_i']
  Integrator1 : Integrator  InitialCondition=[lambda_i; D_fv_i']
  Matrix Multiply : Product
  Matrix Multiply1 : Product  Multiplication=Matrix(*)
  Projection operator : MATLAB Function  Commented=on  TreatAsAtomicUnit=on
  Scope : Scope
  Scope1 : Scope
  Switch : Switch  Criteria=u2 > Threshold  Threshold=0.5  SaturateOnIntegerOverflow=off  InputSameDT=off
  theta_a : Outport
  wires:
  Constant/1 -> Gain/1
  Gain/1 -> Matrix Multiply/1
  phia/1 -> Matrix Multiply/2
  Matrix Multiply/1 -> Matrix Multiply1/1
  ev/1 -> Matrix Multiply1/2
  Matrix Multiply1/1 -> Integrator/1, Projection operator/2(y)
  Integrator/1 -> Switch/3
  Projection operator/2(y_proj) -> Integrator1/1
  Integrator1/1 -> Projection operator/1(theta_a_hat), Switch/1
  Constant1/1 -> Switch/2
  Switch/1 -> theta_a/1
  Projection operator/1(f) -> Scope/1
  Projection operator/3(ygrad) -> Scope1/1

== system UAV_Task3/POSITION + ADAPTIVE CONTROLLER/Subsystem1/Subsystem2 ==
  lambda_mx : Inport
  ub : Inport  Port=2
  phipT : Inport  Port=3
  thetap_hat : Inport  Port=4
  Constant : Constant  Value=eye(3)
  Invert 3x3 Matrix : aerolibutil/Invert  3x3 Matrix
  Matrix Multiply : Product  Multiplication=Matrix(*)
  Matrix Multiply1 : Product  Multiplication=Matrix(*)
  Matrix Multiply2 : Product  Multiplication=Matrix(*)
  Sum : Sum  Inputs=|+-
  Sum1 : Sum  Inputs=+-
  ua : Outport
  wires:
  lambda_mx/1 -> Invert 3x3 Matrix/1
  Invert 3x3 Matrix/1 -> Matrix Multiply1/1, Sum/1
  Constant/1 -> Sum/2
  Sum/1 -> Matrix Multiply/1
  ub/1 -> Matrix Multiply/2
  Matrix Multiply/1 -> Sum1/1
  phipT/1 -> Matrix Multiply1/2
  Matrix Multiply1/1 -> Matrix Multiply2/1
  thetap_hat/1 -> Matrix Multiply2/2
  Matrix Multiply2/1 -> Sum1/2
  Sum1/1 -> ua/1

== system UAV_Task3/Position Controller/Adaptive Augmentation/Predictor (x_p_hat) dynamics ==
  Lambda_hat : Inport
  u : Inport  Port=2
  phi_p : Inport  Port=3
  theta_p_hat : Inport  Port=4
  x_p : Inport  Port=5
  Add : Sum
  Constant : Constant  Value=par.g*par.e_3
  Gain : Gain  Gain=B_p  Multiplication=Matrix(K*u)
  Gain1 : Gain  Gain=L
  Gain2 : Gain  Gain=gravityInAdaptiveController
  Gain3 : Gain
  Integrator : Integrator  InitialCondition=vb_0
  Matrix Multiply : Product
  Matrix Multiply1 : Product  Multiplication=Matrix(*)
  Reshape : Reshape  OutputDimensionality=Column vector (2-D)
  Reshape1 : Reshape  OutputDimensionality=Column vector (2-D)
  Reshape2 : Reshape  OutputDimensionality=Column vector (2-D)
  Scope : Scope
  Scope1 : Scope
  Sum : Sum  Inputs=+++
  Sum1 : Sum  Inputs=-+|
  Transpose : Math  Operator=transpose
  x_p_hat : Outport
  wires:
  Lambda_hat/1 -> Matrix Multiply/1
  phi_p/1 -> Transpose/1
  theta_p_hat/1 -> Matrix Multiply1/2
  Gain/1 -> Reshape1/1
  Gain1/1 -> Reshape/1
  x_p/1 -> Scope1/1, Sum1/2
  Sum1/1 -> Gain1/1
  Integrator/1 -> Scope/1, Sum1/1, x_p_hat/1
  Reshape/1 -> Sum/1  "prediction_error"
  Reshape1/1 -> Sum/2  "dynamics"
  Reshape2/1 -> Sum/3  "gravity"
  Constant/1 -> Gain2/1
  Transpose/1 -> Matrix Multiply1/1
  u/1 -> Matrix Multiply/2
  Gain2/1 -> Gain3/1
  Gain3/1 -> Reshape2/1
  Matrix Multiply1/1 -> Add/2
  Add/1 -> Gain/1
  Matrix Multiply/1 -> Add/1
  Sum/1 -> Integrator/1

== system UAV_Task3/Position Controller/Adaptive Augmentation/Subsystem ==
  Lambda_hat : Inport
  u_b : Inport  Port=2
  phi_p : Inport  Port=3
  theta_p_hat : Inport  Port=4
  Constant : Constant  Value=eye(3,3)
  Gain : Gain  Commented=through  Gain=-1
  Gain1 : Gain
  Inverse : MATLAB Function  TreatAsAtomicUnit=on
  Product : Product  Multiplication=Matrix(*)
  Product1 : Product  Inputs=3  Multiplication=Matrix(*)
  Subtract : Sum  Inputs=-+
  Subtract1 : Sum  Inputs=+-
  Transpose : Math  Operator=transpose
  u_a : Outport
  wires:
  Lambda_hat/1 -> Inverse/1(u)
  Inverse/1(y) -> Product1/1, Subtract/2
  Constant/1 -> Subtract/1
  Subtract/1 -> Product/1
  u_b/1 -> Product/2
  Product/1 -> Gain1/1
  Subtract1/1 -> u_a/1
  phi_p/1 -> Transpose/1
  Transpose/1 -> Gain/1
  theta_p_hat/1 -> Product1/3
  Product1/1 -> Subtract1/2
  Gain/1 -> Product1/2
  Gain1/1 -> Subtract1/1

== system UAV_Task3/Position Controller/Adaptive Augmentation/phi_a ==
  u : Inport
  phi_p : Inport  Port=2
  Matrix Concatenate : Concatenate  Mode=Multidimensional array
  Scope : Scope
  Transpose : Math  Operator=transpose
  phi_a : Outport
  wires:
  Matrix Concatenate/1 -> Scope/1, phi_a/1
  u/1 -> Transpose/1
  phi_p/1 -> Matrix Concatenate/2
  Transpose/1 -> Matrix Concatenate/1

== system UAV_Task3/Position Controller/Adaptive Augmentation/phi_p ==
  x_p : Inport
  Create Diagonal Matrix : matrix_library/Create Diagonal Matrix
  Gain : Gain  Gain=-1
  phi_p : Outport
  wires:
  x_p/1 -> Gain/1
  Gain/1 -> Create Diagonal Matrix/1
  Create Diagonal Matrix/1 -> phi_p/1

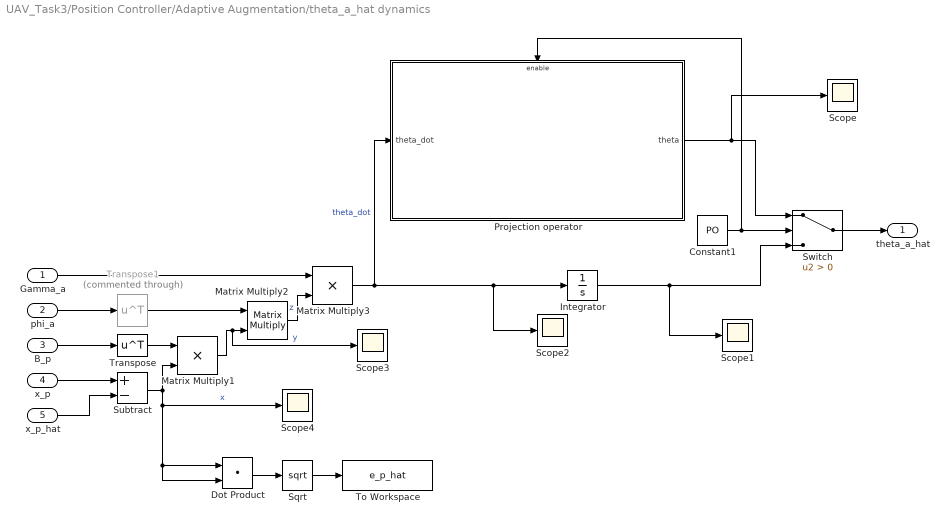
== system UAV_Task3/Position Controller/Adaptive Augmentation/theta_a_hat dynamics ==
  Gamma_a : Inport
  phi_a : Inport  Port=2
  B_p : Inport  Port=3
  x_p : Inport  Port=4
  x_p_hat : Inport  Port=5
  Constant1 : Constant  Value=PO
  Dot Product : DotProduct  OutDataTypeStr=Inherit: Inherit via internal rule
  Integrator : Integrator  InitialCondition=[lambda_0; theta_0]
  Matrix Multiply1 : Product
  Matrix Multiply2 : Product  Multiplication=Matrix(*)
  Matrix Multiply3 : Product
  Projection operator : Subsystem
  Scope{,1..4} (5 alike) : Scope
  Sqrt : Sqrt
  Subtract : Sum  Inputs=+-
  Switch : Switch  Criteria=u2 > Threshold  SaturateOnIntegerOverflow=off  InputSameDT=off
  To Workspace : ToWorkspace  VariableName=e_p_hat  SaveFormat=Timeseries  SampleTime=-1
  Transpose : Math  Operator=transpose
  Transpose1 : Math  Commented=through  Operator=transpose
  theta_a_hat : Outport
  wires:
  x_p_hat/1 -> Subtract/2
  B_p/1 -> Transpose/1
  Subtract/1 -> Scope4/1, Dot Product/2, Dot Product/1, Matrix Multiply1/2  "x"
  Transpose/1 -> Matrix Multiply1/1
  phi_a/1 -> Transpose1/1
  Matrix Multiply1/1 -> Scope3/1, Matrix Multiply2/2  "y"
  Gamma_a/1 -> Matrix Multiply3/1
  Matrix Multiply2/1 -> Matrix Multiply3/2  "z"
  Matrix Multiply3/1 -> Projection operator/1(theta_dot), Scope2/1, Integrator/1  "theta_dot"
  x_p/1 -> Subtract/1
  Constant1/1 -> Switch/2, Projection operator/Enable
  Integrator/1 -> Scope1/1, Switch/3
  Switch/1 -> theta_a_hat/1
  Projection operator/1(theta) -> Scope/1, Switch/1
  Dot Product/1 -> Sqrt/1
  Sqrt/1 -> To Workspace/1
  Transpose1/1 -> Matrix Multiply2/1

== system UAV_Task3/Position Controller/Position controller (Kin)/Subsystem ==
  e_p : Inport
  Action Port : ActionPort  ActionPortLabel=if(u1 == 2)
  Dot Product : DotProduct  OutDataTypeStr=Inherit: Inherit via internal rule
  Sqrt : Sqrt
  Sum of Elements : Sum  Inputs=+
  To Workspace : ToWorkspace  VariableName=posRMS  SaveFormat=Timeseries  SampleTime=-1
  wires:
  e_p/1 -> Dot Product/2, Dot Product/1
  Dot Product/1 -> Sum of Elements/1
  Sum of Elements/1 -> Sqrt/1
  Sqrt/1 -> To Workspace/1

== system UAV_Task3/Position Controller/Subsystem1/Subsystem ==
  v : Inport
  phipT : Inport  Port=2
  lambda_hat : Inport  Port=3
  u : Inport  Port=4
  thetap_hat : Inport  Port=5
  Constant : Constant  Value=[0 0 g]
  Gain : Gain  Gain=1/UAV.m
  Gain1 : Gain  Gain=L
  Integrator : Integrator  InitialCondition=vb_0
  Matrix Multiply : Product  Multiplication=Matrix(*)
  Matrix Multiply1 : Product  Multiplication=Matrix(*)
  Sum : Sum  Inputs=+++
  Sum1 : Sum
  Sum2 : Sum  Inputs=|+-
  v_hat : Outport
  ev : Outport  Port=2
  wires:
  lambda_hat/1 -> Matrix Multiply/1
  u/1 -> Matrix Multiply/2
  phipT/1 -> Matrix Multiply1/1
  thetap_hat/1 -> Matrix Multiply1/2
  Matrix Multiply1/1 -> Sum1/1
  Matrix Multiply/1 -> Sum1/2
  Sum1/1 -> Gain/1
  Constant/1 -> Sum/1
  Gain/1 -> Sum/2
  Sum/1 -> Integrator/1
  Integrator/1 -> Sum2/2, v_hat/1
  v/1 -> Sum2/1
  Sum2/1 -> ev/1, Gain1/1
  Gain1/1 -> Sum/3

== system UAV_Task3/Position Controller/Subsystem1/Subsystem1 ==
  phia : Inport
  ev : Inport  Port=2
  Constant : Constant  Value=Gamma_a_scalar
  Constant1 : Constant  Value=projection_operator
  Gain : Gain  Gain=1/UAV.m
  Integrator : Integrator  InitialCondition=[lambda_i; D_fv_i']
  Integrator1 : Integrator  InitialCondition=[lambda_i; D_fv_i']
  Matrix Multiply : Product
  Matrix Multiply1 : Product  Multiplication=Matrix(*)
  Projection operator : MATLAB Function  Commented=on  TreatAsAtomicUnit=on
  Reshape : Reshape  OutputDimensionality=Column vector (2-D)
  Scope : Scope
  Scope1 : Scope
  Switch : Switch  Criteria=u2 > Threshold  Threshold=0.5  SaturateOnIntegerOverflow=off  InputSameDT=off
  theta_a : Outport
  wires:
  Constant/1 -> Reshape/1
  Gain/1 -> Matrix Multiply/1
  phia/1 -> Matrix Multiply/2
  Matrix Multiply/1 -> Matrix Multiply1/1
  ev/1 -> Matrix Multiply1/2
  Matrix Multiply1/1 -> Integrator/1, Projection operator/2(y)
  Integrator/1 -> Switch/3
  Projection operator/2(y_proj) -> Integrator1/1
  Integrator1/1 -> Projection operator/1(theta_a_hat), Switch/1
  Constant1/1 -> Switch/2
  Switch/1 -> theta_a/1
  Projection operator/1(f) -> Scope/1
  Projection operator/3(ygrad) -> Scope1/1
  Reshape/1 -> Gain/1

== system UAV_Task3/Position Controller/Subsystem1/Subsystem2 ==
  lambda_mx : Inport
  ub : Inport  Port=2
  phipT : Inport  Port=3
  thetap_hat : Inport  Port=4
  Constant : Constant  Value=eye(3)
  Invert 3x3 Matrix : aerolibutil/Invert  3x3 Matrix
  Matrix Multiply : Product  Multiplication=Matrix(*)
  Matrix Multiply1 : Product  Multiplication=Matrix(*)
  Matrix Multiply2 : Product  Multiplication=Matrix(*)
  Sum : Sum  Inputs=|+-
  Sum1 : Sum  Inputs=+-
  ua : Outport
  wires:
  lambda_mx/1 -> Invert 3x3 Matrix/1
  Invert 3x3 Matrix/1 -> Matrix Multiply1/1, Sum/1
  Constant/1 -> Sum/2
  Sum/1 -> Matrix Multiply/1
  ub/1 -> Matrix Multiply/2
  Matrix Multiply/1 -> Sum1/1
  phipT/1 -> Matrix Multiply1/2
  Matrix Multiply1/1 -> Matrix Multiply2/1
  thetap_hat/1 -> Matrix Multiply2/2
  Matrix Multiply2/1 -> Sum1/2
  Sum1/1 -> ua/1

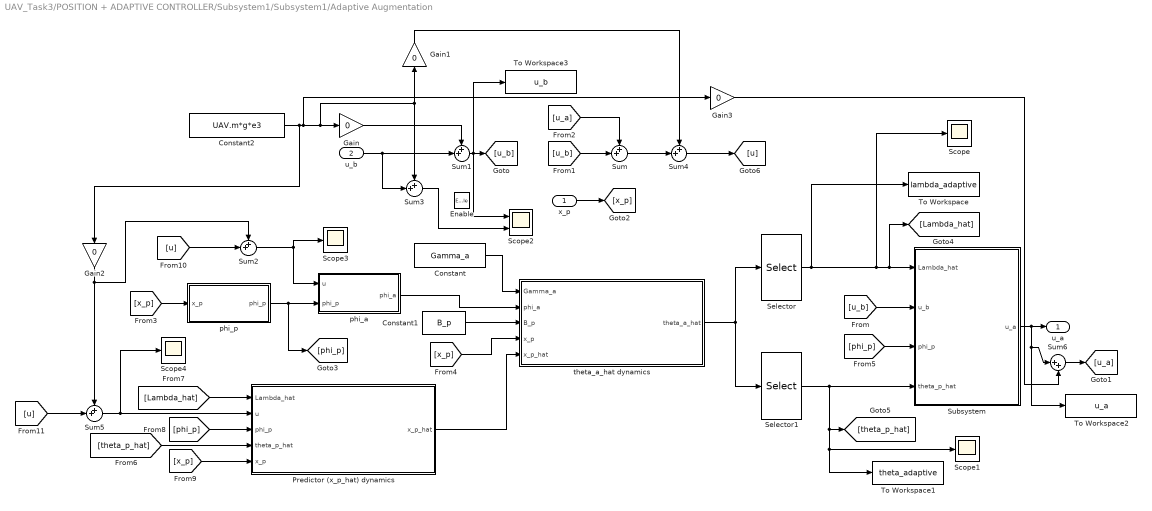
== system UAV_Task3/POSITION + ADAPTIVE CONTROLLER/Subsystem1/Subsystem1/Adaptive Augmentation ==
  x_p : Inport
  u_b : Inport  Port=2
  Enable : EnablePort
  Constant : Constant  Value=Gamma_a
  Constant1 : Constant  Value=B_p
  Constant2 : Constant  Value=UAV.m*g*e3
  Gain{,1..3} (4 alike) : Gain  Gain=0
  Predictor (x_p_hat) dynamics : Subsystem
  Scope{,1,3..4} (4 alike) : Scope
  Scope2 : Scope  NumInputPorts=2
  Selector : Selector  InputPortWidth=4  IndexOptions=Index vector (dialog)  Indices=[1]  OutputSizes=1
  Selector1 : Selector  InputPortWidth=4  IndexOptions=Index vector (dialog)  Indices=[2 3 4]  OutputSizes=1
  Subsystem : Subsystem
  Sum{,1..5} (6 alike) : Sum  Inputs=++|
  Sum6 : Sum  Inputs=|++
  To Workspace : ToWorkspace  VariableName=lambda_adaptive  SaveFormat=Timeseries  SampleTime=-1
  To Workspace1 : ToWorkspace  VariableName=theta_adaptive  SaveFormat=Timeseries  SampleTime=-1
  To Workspace2 : ToWorkspace  VariableName=u_a  SaveFormat=Timeseries  SampleTime=-1
  To Workspace3 : ToWorkspace  VariableName=u_b  SaveFormat=Timeseries  SampleTime=-1
  phi_a : Subsystem
  phi_p : Subsystem
  theta_a_hat dynamics : Subsystem
  u_a : Outport
  wires:
  Selector1/1 -> Scope1/1, To Workspace1/1, [theta_p_hat], Subsystem/4(theta_p_hat)
  theta_a_hat dynamics/1(theta_a_hat) -> Selector/1, Selector1/1
  Constant/1 -> theta_a_hat dynamics/1(Gamma_a)
  phi_p/1(phi_p) -> phi_a/2(phi_p), [phi_p]
  [u_b] -> Sum/2
  phi_a/1(phi_a) -> theta_a_hat dynamics/2(phi_a)
  [x_p] -> phi_p/1(x_p)
  [x_p] -> theta_a_hat dynamics/4(x_p)
  Constant1/1 -> theta_a_hat dynamics/3(B_p)
  [phi_p] -> Subsystem/3(phi_p)
  Predictor (x_p_hat) dynamics/1(x_p_hat) -> theta_a_hat dynamics/5(x_p_hat)
  [theta_p_hat] -> Predictor (x_p_hat) dynamics/4(theta_p_hat)
  [Lambda_hat] -> Predictor (x_p_hat) dynamics/1(Lambda_hat)
  [phi_p] -> Predictor (x_p_hat) dynamics/3(phi_p)
  [x_p] -> Predictor (x_p_hat) dynamics/5(x_p)
  x_p/1 -> [x_p]
  [u_a] -> Sum/1
  Selector/1 -> Scope/1, [Lambda_hat], Subsystem/1(Lambda_hat), To Workspace/1
  u_b/1 -> Sum3/2, Sum1/2
  Sum1/1 -> Scope2/1, To Workspace3/1, [u_b]
  [u_b] -> Subsystem/2(u_b)
  Subsystem/1(u_a) -> Sum6/1, To Workspace2/1, u_a/1
  Sum2/1 -> phi_a/1(u), Scope3/1
  [u] -> Sum2/2
  Gain/1 -> Sum1/1
  Sum3/1 -> Scope2/2
  Sum/1 -> Sum4/2
  Sum4/1 -> [u]
  Constant2/1 -> Gain2/1, Gain3/1, Gain1/1, Sum3/1, Gain/1
  Gain1/1 -> Sum4/1
  [u] -> Sum5/2
  Sum5/1 -> Scope4/1, Predictor (x_p_hat) dynamics/2(u)
  Gain2/1 -> Sum2/1, Sum5/1
  Sum6/1 -> [u_a]
  Gain3/1 -> Sum6/2

== system UAV_Task3/Position Controller/Adaptive Augmentation/theta_a_hat dynamics/Projection operator ==
  theta_dot : Inport
  Enable : EnablePort
  Constant : Constant  Value=lambda_0
  Constant3 : Constant  Value=theta_0(1)
  Constant4 : Constant  Value=theta_0(2)
  Constant5 : Constant  Value=theta_0(3)
  Demux : Demux
  Integrator{1,4..6} (4 alike) : Integrator
  MATLAB Function : MATLAB Function  TreatAsAtomicUnit=on
  MATLAB Function3 : MATLAB Function  TreatAsAtomicUnit=on
  MATLAB Function4 : MATLAB Function  TreatAsAtomicUnit=on
  MATLAB Function5 : MATLAB Function  TreatAsAtomicUnit=on
  Mux : Mux
  Sum{,3..5} (4 alike) : Sum  Inputs=|++
  theta : Outport
  wires:
  MATLAB Function/1(y_proj) -> Integrator1/1
  Sum/1 -> MATLAB Function/1(theta), Mux/1
  Integrator1/1 -> Sum/1
  Constant/1 -> Sum/2
  Demux/1 -> MATLAB Function/2(theta_dot)
  theta_dot/1 -> Demux/1
  Constant3/1 -> Sum3/2
  MATLAB Function3/1(y_proj) -> Integrator4/1
  Sum3/1 -> Mux/2, MATLAB Function3/1(theta)
  Integrator4/1 -> Sum3/1
  Demux/2 -> MATLAB Function3/2(theta_dot)
  Constant4/1 -> Sum4/2
  MATLAB Function4/1(y_proj) -> Integrator5/1
  Sum4/1 -> Mux/3, MATLAB Function4/1(theta)
  Integrator5/1 -> Sum4/1
  Demux/3 -> MATLAB Function4/2(theta_dot)
  Constant5/1 -> Sum5/2
  MATLAB Function5/1(y_proj) -> Integrator6/1
  Sum5/1 -> MATLAB Function5/1(theta), Mux/4
  Integrator6/1 -> Sum5/1
  Demux/4 -> MATLAB Function5/2(theta_dot)
  Mux/1 -> theta/1
